simulink model "back_calculation"  (R2022a)
settings: Solver=VariableStepAuto  StartTime=0.0  StopTime=10.0  RelTol=1e-3
settings Model: Creator=souza  LastModifiedBy=souza

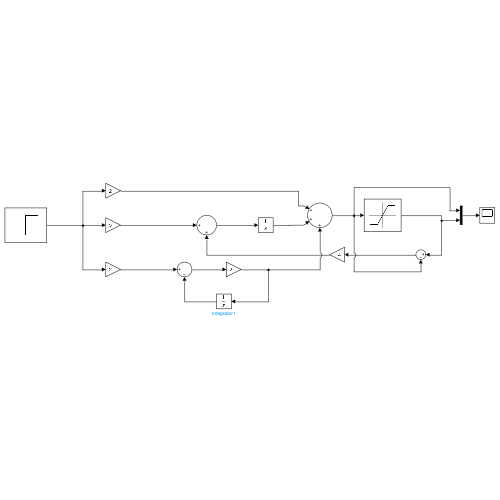
[thumbnail: Simulink's stored preview of the top-level diagram]
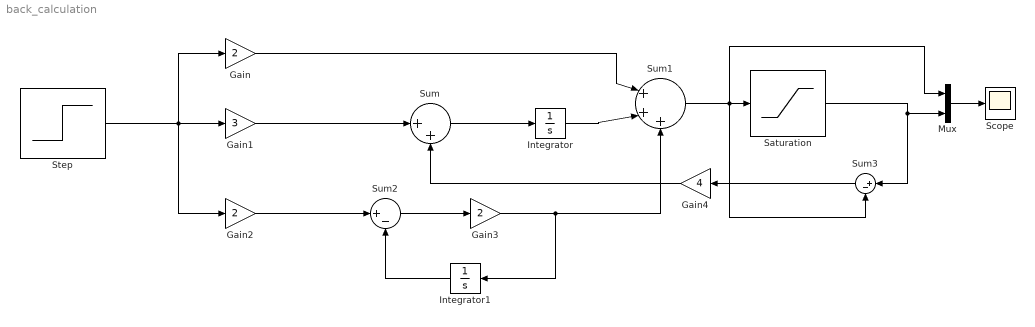
== system back_calculation ==
  Gain : Gain  Gain=2
  Gain1 : Gain  Gain=3
  Gain2 : Gain  Gain=2
  Gain3 : Gain  Gain=2
  Gain4 : Gain  Gain=4
  Integrator : Integrator
  Integrator1 : Integrator
  Mux : Mux  Inputs=2
  Saturation : Saturate  UpperLimit=5  LowerLimit=0
  Scope : Scope
  Step : Step  After=5  SampleTime=0
  Sum : Sum  Inputs=|++
  Sum1 : Sum  Inputs=|+++
  Sum2 : Sum  Inputs=|+-
  Sum3 : Sum  Inputs=|+-
  wires:
  Step/1 -> Gain2/1, Gain/1, Gain1/1
  Gain1/1 -> Sum/1
  Gain/1 -> Sum1/1
  Sum/1 -> Integrator/1
  Integrator/1 -> Sum1/2
  Saturation/1 -> Mux/2, Sum3/1
  Sum1/1 -> Sum3/2, Saturation/1, Mux/1
  Gain2/1 -> Sum2/1
  Integrator1/1 -> Sum2/2
  Sum2/1 -> Gain3/1
  Gain3/1 -> Integrator1/1, Sum1/3
  Sum3/1 -> Gain4/1
  Gain4/1 -> Sum/2
  Mux/1 -> Scope/1
